simulink model "GenTrayectorias"  (R2018a)
settings: Solver=VariableStepAuto  StartTime=0.0  StopTime=2  FixedStep=0.001  RelTol=1e-3
libraries: vrlib x1
settings Model: Creator=Richa  LastModifiedBy=richard
settings CodeAppCC: StateflowObjectComments=on

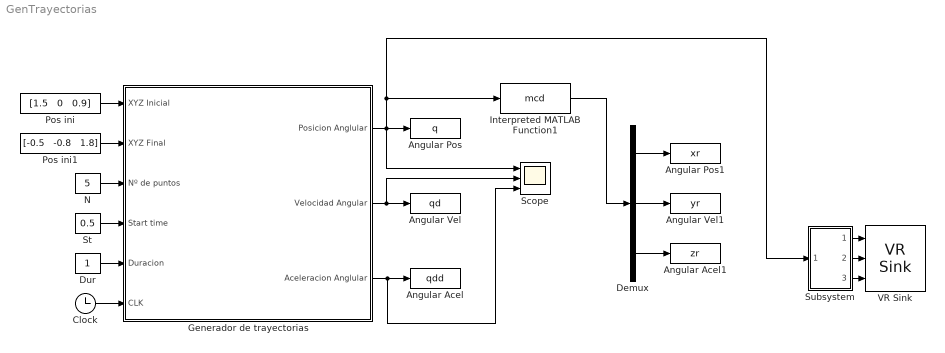
== system GenTrayectorias ==
  Angular Acel : ToWorkspace  VariableName=qdd  SampleTime=-1
  Angular Acel1 : ToWorkspace  VariableName=zr  SampleTime=-1
  Angular Pos : ToWorkspace  VariableName=q  SampleTime=-1
  Angular Pos1 : ToWorkspace  VariableName=xr  SampleTime=-1
  Angular Vel : ToWorkspace  VariableName=qd  SampleTime=-1
  Angular Vel1 : ToWorkspace  VariableName=yr  SampleTime=-1
  Clock : Clock
  Demux : Demux  Outputs=3
  Dur : Constant
  Generador de trayectorias : Subsystem
      mask Display: image('screenshot.png');
  Interpreted MATLAB Function1 : MATLABFcn  MATLABFcn=mcd  OutputDimensions=3
  N : Constant  Value=5
  Pos ini : Constant  Value="[1.5   0   0.9]"
  Pos ini1 : Constant  Value="[-0.5   -0.8   1.8]"
  Scope : Scope  NumInputPorts=3
  St : Constant  Value=0.5
  Subsystem : Subsystem
  VR Sink : vrlib/VR Sink  InstantiateOnLoad=on  SampleTime=0.1  ViewEnable=on  RemoteChange=off  RemoteView=off  FieldsWritten=Rotation_Shoulder.rotation.4.1.1.double#Rotation_Arm.rotation.4.1.1.double#Rotation_ForeArm.rotation.4.1.1.double  WorldFileName=R3GDL.wrl  AutoView=off  VideoDimensions=[]  AllowVariableSize=off
      settings: SourceProductBaseCode=VR
  wires:
  Pos ini/1 -> Generador de trayectorias/1(XYZ Inicial)
  Pos ini1/1 -> Generador de trayectorias/2(XYZ Final)
  N/1 -> Generador de trayectorias/3(Nº de puntos)
  St/1 -> Generador de trayectorias/4(Start time)
  Dur/1 -> Generador de trayectorias/5(Duracion)
  Clock/1 -> Generador de trayectorias/6(CLK)
  Generador de trayectorias/2(Velocidad Angular) -> Scope/2, Angular Vel/1
  Generador de trayectorias/3(Aceleracion Anglular) -> Scope/3, Angular Acel/1
  Generador de trayectorias/1(" Posicion Anglular") -> Scope/1, Subsystem/1(In1), Interpreted MATLAB Function1/1, Angular Pos/1
  Interpreted MATLAB Function1/1 -> Demux/1
  Demux/3 -> Angular Acel1/1
  Demux/2 -> Angular Vel1/1
  Demux/1 -> Angular Pos1/1
  Subsystem/1(Out1) -> VR Sink/1
  Subsystem/2(Out2) -> VR Sink/2
  Subsystem/3(Out3) -> VR Sink/3

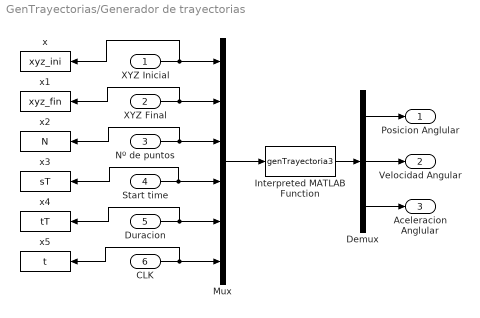
== system GenTrayectorias/Generador de trayectorias ==
  XYZ Inicial : Inport
  XYZ Final : Inport  Port=2
  Nº de puntos : Inport  Port=3
  Start time : Inport  Port=4
  Duracion : Inport  Port=5
  CLK : Inport  Port=6
  Demux : Demux  Outputs=3
  Interpreted MATLAB Function : MATLABFcn  MATLABFcn=genTrayectoria3  OutputDimensions=9
  Mux : Mux  Inputs=6
  x : ToWorkspace  VariableName=xyz_ini  SampleTime=-1
  x1 : ToWorkspace  VariableName=xyz_fin  SampleTime=-1
  x2 : ToWorkspace  VariableName=N  SampleTime=-1
  x3 : ToWorkspace  VariableName=sT  SampleTime=-1
  x4 : ToWorkspace  VariableName=tT  SampleTime=-1
  x5 : ToWorkspace  VariableName=t  SampleTime=-1
  " Posicion Anglular" : Outport  PortDimensions=3
  Velocidad Angular : Outport  Port=2  PortDimensions=3
  Aceleracion Anglular : Outport  Port=3  PortDimensions=3
  wires:
  Demux/3 -> Aceleracion Anglular/1
  Mux/1 -> Interpreted MATLAB Function/1
  Nº de puntos/1 -> x2/1, Mux/3
  CLK/1 -> x5/1, Mux/6
  Start time/1 -> x3/1, Mux/4
  Interpreted MATLAB Function/1 -> Demux/1
  Duracion/1 -> x4/1, Mux/5
  XYZ Final/1 -> x1/1, Mux/2
  XYZ Inicial/1 -> x/1, Mux/1
  Demux/1 -> " Posicion Anglular"/1
  Demux/2 -> Velocidad Angular/1

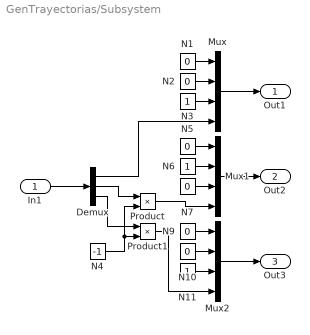
== system GenTrayectorias/Subsystem ==
  In1 : Inport
  Demux : Demux  Outputs=3
  Mux : Mux
  Mux1 : Mux
  Mux2 : Mux
  N{1..2,5,7,9..10} (6 alike) : Constant  Value=0
  N11 : Constant
  N3 : Constant
  N4 : Constant  Value=-1
  N6 : Constant
  Product : Product
  Product1 : Product
  Out1 : Outport
  Out2 : Outport  Port=2
  Out3 : Outport  Port=3
  wires:
  N6/1 -> Mux1/2
  N5/1 -> Mux1/1
  Product/1 -> Mux1/4
  N10/1 -> Mux2/2
  Mux2/1 -> Out3/1
  N9/1 -> Mux2/1
  N11/1 -> Mux2/3
  N2/1 -> Mux/2
  Mux1/1 -> Out2/1
  N3/1 -> Mux/3
  N1/1 -> Mux/1
  Mux/1 -> Out1/1
  In1/1 -> Demux/1
  Demux/1 -> Mux/4
  Demux/2 -> Product/1
  Demux/3 -> Product1/1
  Product1/1 -> Mux2/4
  N4/1 -> Product1/2, Product/2
  N7/1 -> Mux1/3
